simulink model "State_Machine"  (R2020a)
settings: Solver=VariableStepAuto  StartTime=0.0  StopTime=13  RelTol=1e-3
libraries: simulink_extras x2
settings Model: Creator=ashwin  LastModifiedBy=ashwin

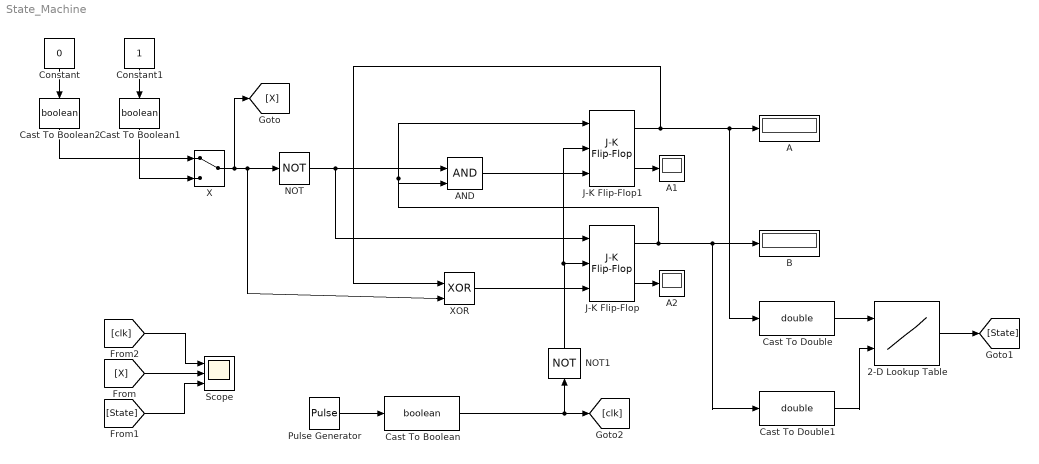
== system State_Machine ==
  2-D Lookup Table : Lookup_n-D  BreakpointsForDimension1=[0, 1]  BreakpointsForDimension2=[0, 1]  Table=reshape([1, 3, 2, 4] , 2, 2)  InternalRulePriority=Speed  RndMeth=Simplest  InputSameDT=on
  A : Display
  A1 : Display
  A2 : Display
  AND : Logic  IconShape=distinctive  AllPortsSameDT=off  OutDataTypeStr=boolean
  B : Display
  Cast To Boolean : DataTypeConversion  OutDataTypeStr=boolean
  Cast To Boolean1 : DataTypeConversion  OutDataTypeStr=boolean
  Cast To Boolean2 : DataTypeConversion  OutDataTypeStr=boolean
  Cast To Double : DataTypeConversion  OutDataTypeStr=double
  Cast To Double1 : DataTypeConversion  OutDataTypeStr=double
  Constant : Constant  Value=0
  Constant1 : Constant
  J-K Flip-Flop : simulink_extras/Flip Flops/J-K Flip-Flop  initial_condition=0
  J-K Flip-Flop1 : simulink_extras/Flip Flops/J-K Flip-Flop  initial_condition=0
  NOT : Logic  Operator=NOT  IconShape=distinctive  AllPortsSameDT=off  OutDataTypeStr=boolean
  NOT1 : Logic  Operator=NOT  IconShape=distinctive  AllPortsSameDT=off  OutDataTypeStr=boolean
  Pulse Generator : DiscretePulseGenerator  PulseType=Time based  PulseWidth=50
  Scope : Scope  NumInputPorts=3
  X : ManualSwitch
  XOR : Logic  Operator=XOR  IconShape=distinctive  AllPortsSameDT=off  OutDataTypeStr=boolean
  wires:
  AND/1 -> J-K Flip-Flop1/3
  XOR/1 -> J-K Flip-Flop/3
  X/1 -> [X], XOR/2, NOT/1
  Constant/1 -> Cast To Boolean2/1
  Constant1/1 -> Cast To Boolean1/1
  J-K Flip-Flop/1 -> Cast To Double1/1, B/1, AND/2, J-K Flip-Flop1/1
  Pulse Generator/1 -> Cast To Boolean/1
  Cast To Boolean/1 -> NOT1/1, [clk]
  J-K Flip-Flop1/1 -> Cast To Double/1, A/1, XOR/1
  NOT/1 -> J-K Flip-Flop/1, AND/1
  [State] -> Scope/3
  [X] -> Scope/2
  J-K Flip-Flop1/2 -> A1/1
  J-K Flip-Flop/2 -> A2/1
  Cast To Double/1 -> 2-D Lookup Table/1
  Cast To Double1/1 -> 2-D Lookup Table/2
  2-D Lookup Table/1 -> [State]
  [clk] -> Scope/1
  Cast To Boolean1/1 -> X/2
  Cast To Boolean2/1 -> X/1
  NOT1/1 -> J-K Flip-Flop1/2, J-K Flip-Flop/2
